simulink model "lab2"  (R2020b)
settings: Solver=VariableStepAuto  StartTime=0.0  StopTime=10.0  RelTol=1e-3
settings Model: Creator=payal  LastModifiedBy=payal

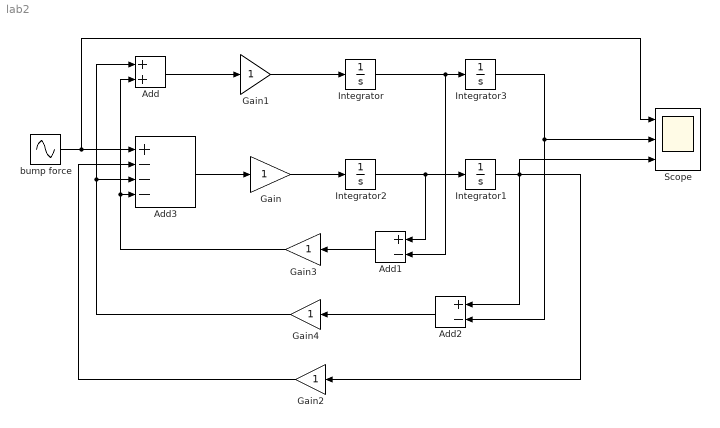
== system lab2 ==
  Add : Sum
  Add1 : Sum  Inputs=+-
  Add2 : Sum  Inputs=+-
  Add3 : Sum  Inputs=+---
  Gain{,1..4} (5 alike) : Gain
  Integrator{,1..3} (4 alike) : Integrator
  Scope : Scope  NumInputPorts=3
  bump force : Sin  SampleTime=0
  wires:
  bump force/1 -> Add3/1, Scope/1
  Add3/1 -> Gain/1
  Gain/1 -> Integrator2/1
  Integrator2/1 -> Add1/1, Integrator1/1
  Add/1 -> Gain1/1
  Gain1/1 -> Integrator/1
  Integrator/1 -> Add1/2, Integrator3/1
  Add1/1 -> Gain3/1
  Add2/1 -> Gain4/1
  Gain3/1 -> Add/2, Add3/4
  Gain4/1 -> Add/1, Add3/3
  Gain2/1 -> Add3/2
  Integrator1/1 -> Gain2/1, Add2/1, Scope/3
  Integrator3/1 -> Add2/2, Scope/2
